simulink model "humidifier"  (R2020b)
settings: Solver=VariableStepAuto  StartTime=0.0  StopTime=10.0  RelTol=1e-3
undefined symbols (not defined in the file): densAir
settings Model: Creator=xinbo  LastModifiedBy=xinbo

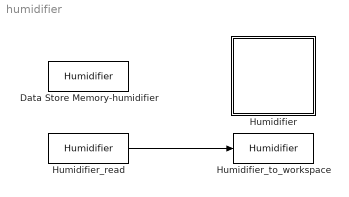
== system humidifier ==
  Data Store Memory-humidifier : DataStoreMemory  DataStoreName=Humidifier  ReadBeforeWriteMsg=warning  WriteAfterWriteMsg=warning  WriteAfterReadMsg=warning  ShowAdditionalParam=off
  Humidifier : Subsystem
      mask Display: image('/Users/xinbo/E/paper3/program_clean/digital_twin/images/humidifier.png'); % Use "Edit Image" on toolstrip to change.
  Humidifier_read : DataStoreRead  DataStoreName=Humidifier
  Humidifier_to_workspace : ToWorkspace  VariableName=Humidifier  SampleTime=-1
      settings: Save2DSignal=2-D array (concatenate along first dimension)
  wires:
  Humidifier_read/1 -> Humidifier_to_workspace/1

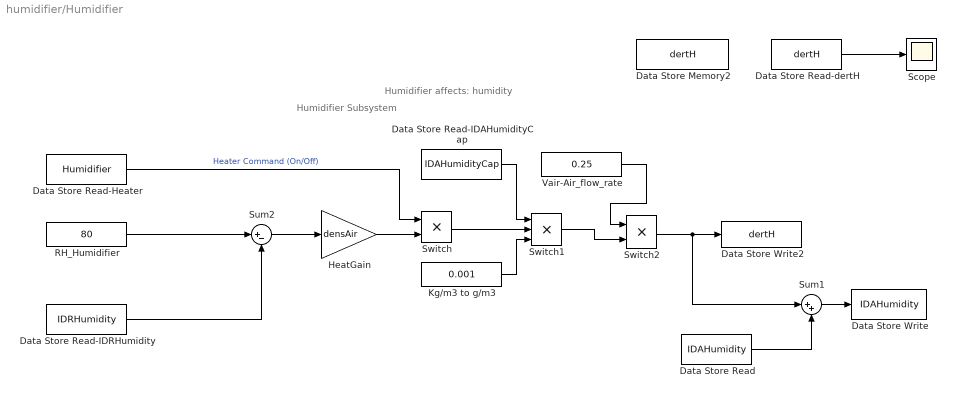
== system humidifier/Humidifier ==
  note: Humidifier affects:
      | humidity
  note: Humidifier
      |  Subsystem
  " Switch" : Product  RndMeth=Zero
  " Switch1" : Product  Inputs=3  RndMeth=Zero
  " Switch2" : Product  RndMeth=Zero
  Data Store Read : DataStoreRead  DataStoreName=IDAHumidity
  Data Store Read-Heater : DataStoreRead  DataStoreName=Humidifier
  Data Store Read-IDAHumidityCap : DataStoreRead  DataStoreName=IDAHumidityCap
  Data Store Read-IDRHumidity : DataStoreRead  DataStoreName=IDRHumidity
  Data Store Read-dertH : DataStoreRead  DataStoreName=dertH
  Data Store Write : DataStoreWrite  DataStoreName=IDAHumidity
  Data Store Write2 : DataStoreWrite  DataStoreName=dertH
  Data Store Memory2 : DataStoreMemory  DataStoreName=dertH  ReadBeforeWriteMsg=warning  WriteAfterWriteMsg=warning  WriteAfterReadMsg=warning  ShowAdditionalParam=off
  HeatGain : Gain  Gain=densAir
  Kg/m3 to g/m3 : Constant  Value=0.001
  RH_Humidifier : Constant  Value=80
  Scope : Scope
  Sum1 : Sum  Inputs=|++
  Sum2 : Sum  Inputs=|+-
  Vair-Air_flow_rate : Constant  Value=0.25
  wires:
  Data Store Read-Heater/1 -> " Switch"/1  "Heater Command (On/Off)"
  Sum2/1 -> HeatGain/1
  RH_Humidifier/1 -> Sum2/1
  HeatGain/1 -> " Switch"/2
  " Switch"/1 -> " Switch1"/2
  Data Store Read-IDRHumidity/1 -> Sum2/2
  Data Store Read-IDAHumidityCap/1 -> " Switch1"/1
  Kg/m3 to g/m3/1 -> " Switch1"/3
  " Switch1"/1 -> " Switch2"/2
  Vair-Air_flow_rate/1 -> " Switch2"/1
  " Switch2"/1 -> Sum1/1, Data Store Write2/1
  Sum1/1 -> Data Store Write/1
  Data Store Read-dertH/1 -> Scope/1
  Data Store Read/1 -> Sum1/2
